simulink model "Subsystem"  (R2020b)
settings: Solver=VariableStepAuto  StartTime=0.0  StopTime=10.0  RelTol=1e-3
settings Model: Creator=vijay jagtap  LastModifiedBy=vijay jagtap
settings DataIOCC: SaveOutput=off  SaveTime=off

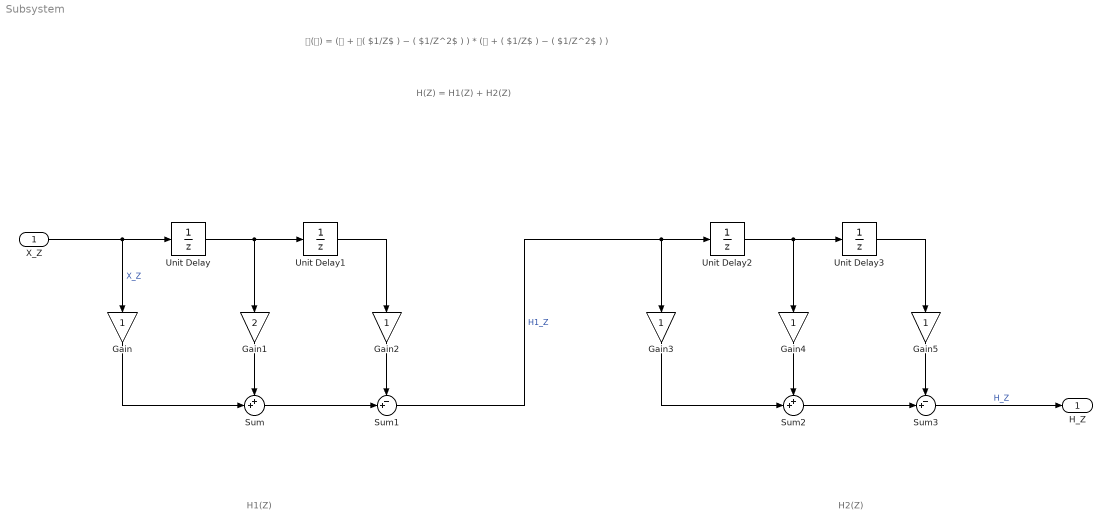
== system Subsystem ==
  note: H2(Z)
  note: 𝐇(𝐳) = (𝟏 + 𝟐( $1/Z$ ) − ( $1/Z^2$ ) ) * (𝟏 + ( $1/Z$ ) − ( $1/Z^2$ ) )
  note: H1(Z)
  note: H(Z) = H1(Z) + H2(Z)
  X_Z : Inport  OutDataTypeStr=double  PortDimensions=1  SampleTime=[0,1]
  Gain{,2..5} (5 alike) : Gain
  Gain1 : Gain  Gain=2
  Sum : Sum  Inputs=++|
  Sum1 : Sum  Inputs=-+|
  Sum2 : Sum  Inputs=++|
  Sum3 : Sum  Inputs=-+|
  Unit Delay{,1..3} (4 alike) : UnitDelay  SampleTime=-1  HasFrameUpgradeWarning=on
  H_Z : Outport  OutDataTypeStr=double  PortDimensions=1  SampleTime=[0,1]
  wires:
  Sum2/1 -> Sum3/2
  Unit Delay3/1 -> Gain5/1
  Unit Delay2/1 -> Unit Delay3/1, Gain4/1
  Sum1/1 -> Unit Delay2/1, Gain3/1  "H1_Z"
  Gain3/1 -> Sum2/2
  Gain5/1 -> Sum3/1
  Gain4/1 -> Sum2/1
  Sum3/1 -> H_Z/1  "H_Z"
  Gain2/1 -> Sum1/1
  Gain/1 -> Sum/2
  X_Z/1 -> Unit Delay/1, Gain/1  "X_Z"
  Unit Delay/1 -> Unit Delay1/1, Gain1/1
  Sum/1 -> Sum1/2
  Unit Delay1/1 -> Gain2/1
  Gain1/1 -> Sum/1
